simulink model "raspberry_net_test_R2021a"  (R2021a)
settings: Solver=FixedStepAuto  StartTime=0.0  StopTime=20  RelTol=1e-3  EnableMultiTasking=on
libraries: deeplib x1
settings Model: SimulationMode=external  Creator=vic-b  LastModifiedBy=vic-b
settings SolverCC: PositivePriorityOrder=on
settings OptimizationCC: EnhancedBackFolding=on  PassReuseOutputArgsAs=Individual arguments  ZeroExternalMemoryAtStartup=off  ZeroInternalMemoryAtStartup=off  MaxStackSize=64  OptimizeBlockOrder=speed  DifferentSizesBufferReuse=on  OptimizationCustomize=off  EfficientTunableParamExpr=on
settings DebuggingCC: ParameterTunabilityLossMsg=error
settings HardwareCC: ProdBitPerPointer=32  ProdBitPerSizeT=32  ProdBitPerPtrDiffT=32  ProdLargestAtomicInteger=Long  ProdLargestAtomicFloat=Double  ProdWordSize=32  ProdLongLongMode=on  ProdHWDeviceType=ARM Compatible->ARM Cortex
settings RTWCC: SystemTargetFile=ert.tlc  HardwareBoard=Raspberry Pi  TLCOptions="-aInlineSetEventsForThisBaseRateFcn=TLC_FALSE -aSuppressMultiTaskScheduler=TLC_FALSE  -aRateBasedStepFcn=0"  TemplateMakefile=ert_default_tmf  Toolchain=GNU GCC Embedded Linux  BuildConfiguration=Faster Runs
settings CodeAppCC: ForceParamTrailComments=on  IgnoreCustomStorageClasses=off  OperatorAnnotations=on  SimulinkDataObjDesc=on  SFDataObjDesc=on  InsertBlockDesc=on
settings ERTTargetCC: LogVarNameModifier=none  MatFileLogging=on  SupportVariableSizeSignals=on  ExtModeTransport=2  ExtModeStaticAlloc=on  ExtModeMexFile=ext_xcp  ExtModeIntrfLevel=Level2 - Open

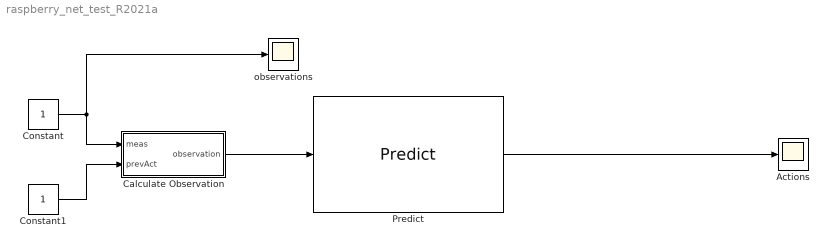
== system raspberry_net_test_R2021a ==
  Actions : Scope
  Calculate Observation : Subsystem
  Constant : Constant
  Constant1 : Constant
  Predict : deeplib/Predict  Network=Network from MAT-file  NetworkFunction=squeezenet  NetworkFilePath=policy.mat  MiniBatchSize=128  InputDataFormats={ '', '' }  Predictions=on  Activations={}  ForceInterpretedSim=off  EnableDLNetwork=on
      settings: SourceProductBaseCode=NN
  observations : Scope
  wires:
  Constant/1 -> observations/1, Calculate Observation/1(meas)
  Constant1/1 -> Calculate Observation/2(prevAct)
  Calculate Observation/1(observation) -> Predict/1
  Predict/1 -> Actions/1

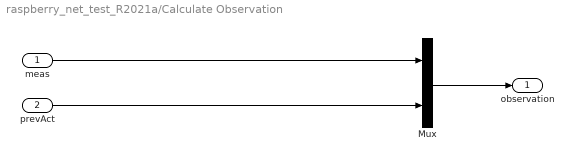
== system raspberry_net_test_R2021a/Calculate Observation ==
  meas : Inport
  prevAct : Inport  Port=2
  Mux : Mux  Inputs=2
  observation : Outport  VectorParamsAs1DForOutWhenUnconnected=off
  wires:
  Mux/1 -> observation/1
  meas/1 -> Mux/1
  prevAct/1 -> Mux/2
